simulink model "LQControl"  (R2015a)
settings: Solver=ode45  StartTime=0.0  StopTime=tijd  RelTol=1e-3
values from neighbouring files (symbols this model uses):
  A = [b1-d1-Y*a 0 0 ... (first row only)    [LQControl.m]    (also in LQControl_script.m; optimalLQControl_script.m = [-(beta1+c) 3*beta2)
  B = [1;0;0]    [LQControl.m]    (also in LQControl_script.m; optimalLQControl_script.m = [-1;0])
  C = [1 0 0 ... (first row only)    [LQControl.m]    (also in LQControl_script.m; optimalLQControl_script.m = [1 0)
  D = [0;0;0]    [LQControl.m]    (also in LQControl_script.m; optimalLQControl_script.m = [0;0])
  K = [-1.9 -980.1 0]*inv(T)    [LQControl.m]    (also in LQControl_script.m)
  k0 = -1.22*10^3    (= -1220)    [LQControl.m]    (also in LQControl_script.m)
  kev = (Y*a*kV)/(d1 - b1 + Y*a)    (= 2222.22222222)    [LQControl.m]    (also in LQControl_script.m)
  s0 = 500    [LQControl.m]    (also in LQControl_script.m)
  v0 = -2.22    [LQControl.m]    (also in LQControl_script.m)
  vev = (a*kV*(b1 - d1))/(d3*(d1 - b1 + Y*a))    (= 22.2222222222)    [LQControl.m]    (also in LQControl_script.m)
settings Model: Creator=Ward  LastModifiedBy=Ward

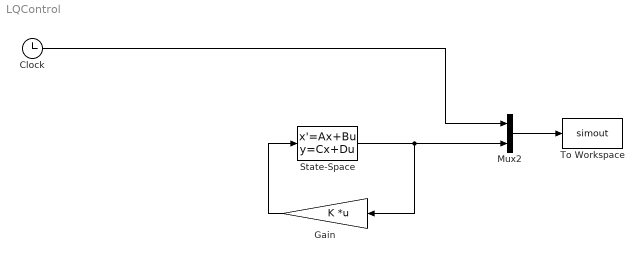
== system LQControl ==
  Clock : Clock
  Gain : Gain  Gain=K  Multiplication=Matrix(K*u)
  Mux2 : Mux  Inputs=2
  State-Space : StateSpace  A=A  B=B  C=C  D=D  X0=[k0-kev;s0;v0-vev]
  To Workspace : ToWorkspace  VariableName=simout  SampleTime=-1
  wires:
  Gain/1 -> State-Space/1
  State-Space/1 -> Gain/1, Mux2/2
  Clock/1 -> Mux2/1
  Mux2/1 -> To Workspace/1
